simulink model "spacecraft"  (R2021a)
settings: Solver=ode45  StartTime=0.0  StopTime=27000  RelTol=1e-12  AbsTol=1e-12
settings Model: Creator=fg7823  LastModifiedBy=fg7823

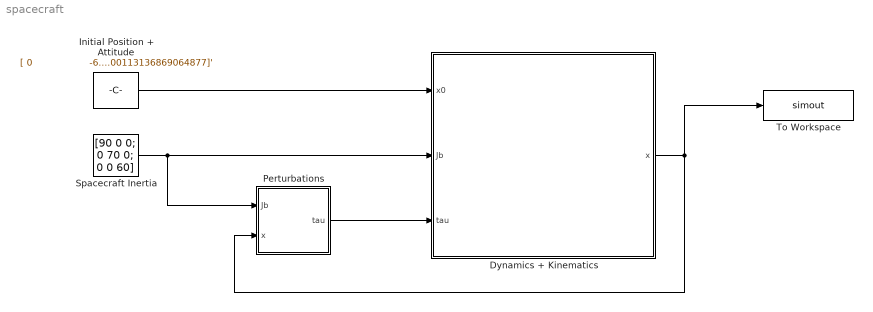
== system spacecraft ==
  Dynamics + Kinematics : Subsystem
  Initial Position + Attitude : Constant  Value=|
      | [ 0
      |                   -6778137
      |                          0
      |           7668.57198272798
      |      0
      |                          0
      |                          0
      |                          0
      |      0
      |                          1
      |       1.74532925199433e-06
      |       1.74532925199433e-06
      |        0.00113136869064877]'
  Perturbations : Subsystem
  Spacecraft Inertia : Constant  Value=[90 0 0; 0 70 0; 0 0 60]
  To Workspace : ToWorkspace  VariableName=simout  SampleTime=-1
  wires:
  Spacecraft Inertia/1 -> Perturbations/1(Jb), Dynamics + Kinematics/2(Jb)
  Initial Position + Attitude/1 -> Dynamics + Kinematics/1(x0)
  Dynamics + Kinematics/1(x) -> To Workspace/1, Perturbations/2(x)
  Perturbations/1(tau) -> Dynamics + Kinematics/3(tau)

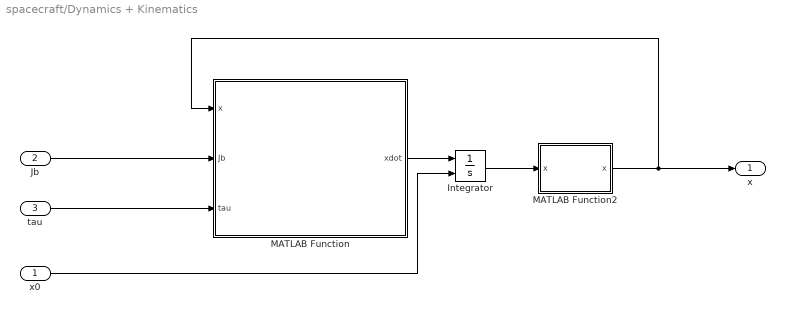
== system spacecraft/Dynamics + Kinematics ==
  x0 : Inport
  Jb : Inport  Port=2
  tau : Inport  Port=3
  Integrator : Integrator  InitialConditionSource=external
  MATLAB Function : MATLAB Function  TreatAsAtomicUnit=on
  MATLAB Function2 : MATLAB Function  TreatAsAtomicUnit=on
  x : Outport
  wires:
  Jb/1 -> MATLAB Function/2(Jb)
  x0/1 -> Integrator/2
  MATLAB Function/1(xdot) -> Integrator/1
  tau/1 -> MATLAB Function/3(tau)
  Integrator/1 -> MATLAB Function2/1("x ")
  MATLAB Function2/1(x) -> x/1, MATLAB Function/1(x)

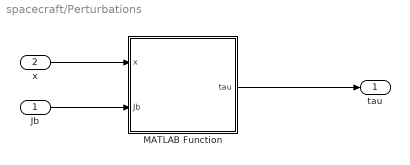
== system spacecraft/Perturbations ==
  Jb : Inport
  x : Inport  Port=2
  MATLAB Function : MATLAB Function  TreatAsAtomicUnit=on
  tau : Outport
  wires:
  x/1 -> MATLAB Function/1(x)
  Jb/1 -> MATLAB Function/2(Jb)
  MATLAB Function/1(tau) -> tau/1

== matlab function spacecraft/Dynamics + Kinematics/MATLAB Function ==
  data: x input; xdot output; Jb input; tau input
function xdot = propagation(x,Jb,tau)
    G           = 6.6743e-11;                    % m3/kgs2
    m_e         = 5.97219e+24;   
    % Unpacking states
    ri          = x(1:3);
    vi          = x(4:6);
    qb_i        = x(7:10);
    wb_bi       = x(11:13);
    xdot        = zeros(13,1);
    % Propagation of position & velocity 
    xdot(1:3)   = vi;
    xdot(4:6)   = -G*m_e*ri/(norm(ri)^3);
    % Propagation of kinematics
    xdot(7:10)  = otimes([wb_bi; 0],qb_i)/2;
    % Propagation of dynamics
    xdot(11:13) = inv(Jb)*(-cross(wb_bi,Jb*wb_bi) + tau);
end

== matlab function spacecraft/Dynamics + Kinematics/MATLAB Function2 ==
  data: x input; x output
function x = normalize(x)
     x(7:10) = x(7:10)/norm(x(7:10));
end

== matlab function spacecraft/Perturbations/MATLAB Function ==
  data: x input; tau output; Jb input
function tau = gravitygradient(x,Jb)
    G    = 6.6743e-11;                    % m3/kgs2
    m_e  = 5.97219e+24;
    n    = sqrt(G*m_e/(400e+3 + 6.3781e+6)^3);
    ri   = x(1:3);
    qb_i = x(7:10);
    rb   = Tq(qb_i)*(-ri);
    db   = rb/norm(rb);
    tau  = 3*cross(db,Jb*db)*n^2;
end
